simulink library "csu_kfo_kalman_filter_output_lib"  (R2015b)
settings: Solver=ode45  StartTime=0.0  StopTime=10.0  RelTol=1e-3
libraries: util_common_lib x4, util_info_lib x2
settings Model: Creator=escrane  LastModifiedBy=Mark Agbayani
settings DataIOCC: SaveFormat=Array
settings DebuggingCC: UnderspecifiedInitializationDetection=Classic  MergeDetectMultiDrivingBlocksExec=none  SolverPrmCheckMsg=warning  StateNameClashWarn=warning
settings HardwareCC: ProdBitPerPointer=32  ProdLargestAtomicFloat=None  ProdIntDivRoundTo=Undefined  ProdEndianess=Unspecified  ProdWordSize=32  ProdHWDeviceType=32-bit Generic
settings GRTTargetCC: GeneratePreprocessorConditionals=Disable all
settings ConfigComp: CovModelRefEnable=Off  CovSFcnEnable=off

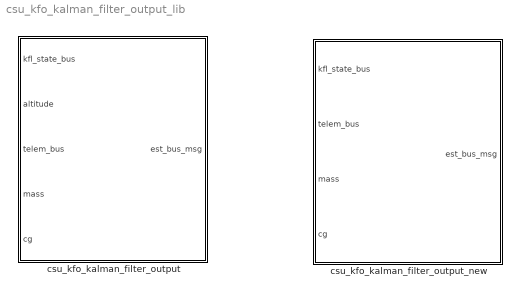
== system csu_kfo_kalman_filter_output_lib ==
  csu_kfo_kalman_filter_output : Subsystem
  csu_kfo_kalman_filter_output_new : Subsystem

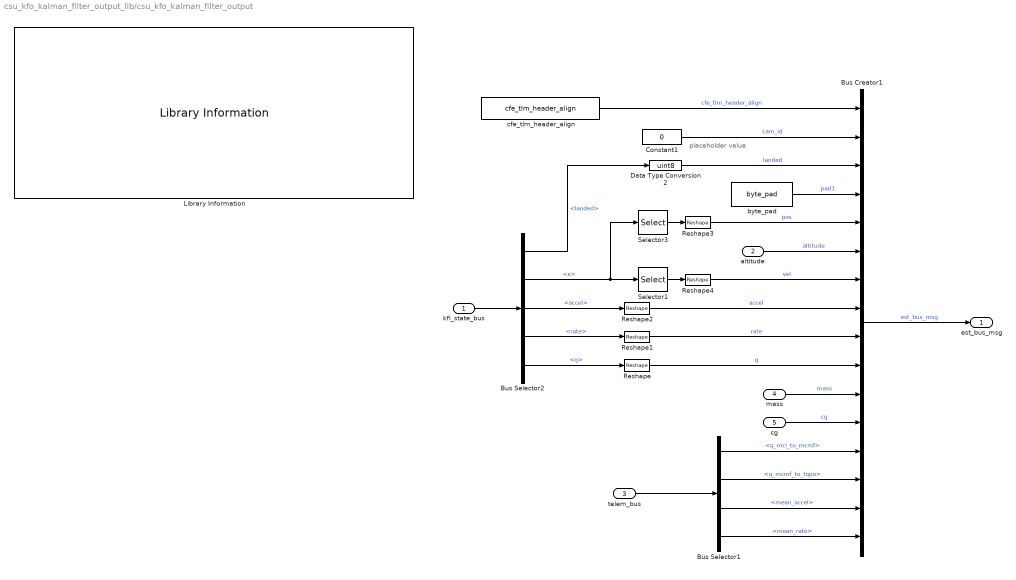
== system csu_kfo_kalman_filter_output_lib/csu_kfo_kalman_filter_output ==
  note: placeholder value
  kfl_state_bus : Inport
  altitude : Inport  Port=2
  telem_bus : Inport  Port=3
  mass : Inport  Port=4
  cg : Inport  Port=5
  Bus Creator1 : BusCreator  Inputs=16  OutDataTypeStr=Bus: est_bus_msg  NonVirtualBus=on
  Bus Selector1 : BusSelector  OutputSignals=q_mci_to_mcmf,q_mcmf_to_topo,mean_accel,mean_rate
  Bus Selector2 : BusSelector  OutputSignals=landed,x,accel,rate,q
  Constant1 : Constant  Value=0  OutDataTypeStr=uint8
  Data Type Conversion2 : DataTypeConversion  OutDataTypeStr=uint8
  Library Information : util_info_lib/Library Information  owner='escrane'
  Reshape{,1..4} (5 alike) : Reshape
  Selector1 : Selector  InputPortWidth=kfl_n_state  IndexOptions=Index vector (dialog)  Indices=kfl_vel_index  OutputSizes=1
  Selector3 : Selector  InputPortWidth=kfl_n_state  IndexOptions=Index vector (dialog)  Indices=kfl_pos_index  OutputSizes=1
  byte_pad : util_common_lib/byte_pad  n_bytes=2
  cfe_tlm_header_align : util_common_lib/cfe_tlm_header_align
  est_bus_msg : Outport
  wires:
  Bus Selector1/4 -> Bus Creator1/16  "<mean_rate>"
  Bus Selector1/3 -> Bus Creator1/15  "<mean_accel>"
  Bus Selector1/1 -> Bus Creator1/13  "<q_mci_to_mcmf>"
  Bus Selector1/2 -> Bus Creator1/14  "<q_mcmf_to_topo>"
  telem_bus/1 -> Bus Selector1/1
  cg/1 -> Bus Creator1/12  "cg"
  mass/1 -> Bus Creator1/11  "mass"
  kfl_state_bus/1 -> Bus Selector2/1
  cfe_tlm_header_align/1 -> Bus Creator1/1  "cfe_tlm_header_align"
  Bus Selector2/1 -> Data Type Conversion2/1  "<landed>"
  byte_pad/1 -> Bus Creator1/4  "pad1"
  Constant1/1 -> Bus Creator1/2  "cam_id"
  Reshape2/1 -> Bus Creator1/8  "accel"
  Bus Creator1/1 -> est_bus_msg/1  "est_bus_msg"
  Bus Selector2/5 -> Reshape/1  "<q>"
  Bus Selector2/4 -> Reshape1/1  "<rate>"
  Bus Selector2/3 -> Reshape2/1  "<accel>"
  Selector1/1 -> Reshape4/1
  Bus Selector2/2 -> Selector1/1, Selector3/1  "<x>"
  Reshape/1 -> Bus Creator1/10  "q"
  Reshape1/1 -> Bus Creator1/9  "rate"
  Reshape4/1 -> Bus Creator1/7  "vel"
  Reshape3/1 -> Bus Creator1/5  "pos"
  Selector3/1 -> Reshape3/1
  Data Type Conversion2/1 -> Bus Creator1/3  "landed"
  altitude/1 -> Bus Creator1/6  "altitude"

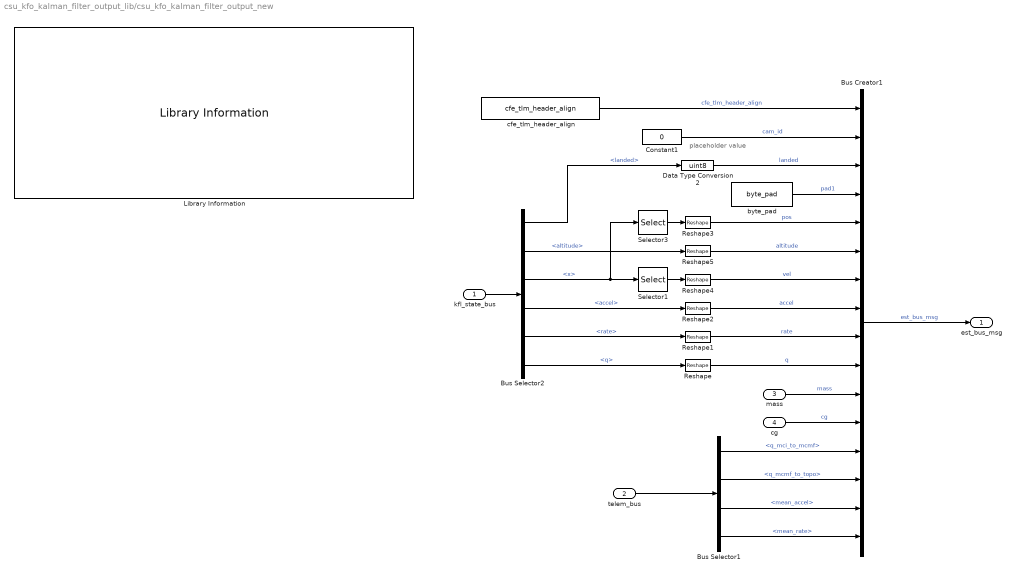
== system csu_kfo_kalman_filter_output_lib/csu_kfo_kalman_filter_output_new ==
  note: placeholder value
  kfl_state_bus : Inport
  telem_bus : Inport  Port=2
  mass : Inport  Port=3
  cg : Inport  Port=4
  Bus Creator1 : BusCreator  Inputs=16  OutDataTypeStr=Bus: est_bus_msg  NonVirtualBus=on
  Bus Selector1 : BusSelector  OutputSignals=q_mci_to_mcmf,q_mcmf_to_topo,mean_accel,mean_rate
  Bus Selector2 : BusSelector  OutputSignals=landed,altitude,x,accel,rate,q
  Constant1 : Constant  Value=0  OutDataTypeStr=uint8
  Data Type Conversion2 : DataTypeConversion  OutDataTypeStr=uint8
  Library Information : util_info_lib/Library Information  owner='escrane'
  Reshape{,1..5} (6 alike) : Reshape
  Selector1 : Selector  InputPortWidth=kfl_n_state  IndexOptions=Index vector (dialog)  Indices=kfl_vel_index  OutputSizes=1
  Selector3 : Selector  InputPortWidth=kfl_n_state  IndexOptions=Index vector (dialog)  Indices=kfl_pos_index  OutputSizes=1
  byte_pad : util_common_lib/byte_pad  n_bytes=2
  cfe_tlm_header_align : util_common_lib/cfe_tlm_header_align
  est_bus_msg : Outport
  wires:
  Reshape5/1 -> Bus Creator1/6  "altitude"
  Bus Selector1/4 -> Bus Creator1/16  "<mean_rate>"
  Bus Selector1/3 -> Bus Creator1/15  "<mean_accel>"
  Bus Selector1/1 -> Bus Creator1/13  "<q_mci_to_mcmf>"
  Bus Selector1/2 -> Bus Creator1/14  "<q_mcmf_to_topo>"
  telem_bus/1 -> Bus Selector1/1
  cg/1 -> Bus Creator1/12  "cg"
  mass/1 -> Bus Creator1/11  "mass"
  kfl_state_bus/1 -> Bus Selector2/1
  cfe_tlm_header_align/1 -> Bus Creator1/1  "cfe_tlm_header_align"
  Bus Selector2/1 -> Data Type Conversion2/1  "<landed>"
  byte_pad/1 -> Bus Creator1/4  "pad1"
  Constant1/1 -> Bus Creator1/2  "cam_id"
  Reshape2/1 -> Bus Creator1/8  "accel"
  Bus Creator1/1 -> est_bus_msg/1  "est_bus_msg"
  Bus Selector2/6 -> Reshape/1  "<q>"
  Bus Selector2/5 -> Reshape1/1  "<rate>"
  Bus Selector2/4 -> Reshape2/1  "<accel>"
  Selector1/1 -> Reshape4/1
  Bus Selector2/3 -> Selector1/1, Selector3/1  "<x>"
  Reshape/1 -> Bus Creator1/10  "q"
  Reshape1/1 -> Bus Creator1/9  "rate"
  Reshape4/1 -> Bus Creator1/7  "vel"
  Reshape3/1 -> Bus Creator1/5  "pos"
  Selector3/1 -> Reshape3/1
  Data Type Conversion2/1 -> Bus Creator1/3  "landed"
  Bus Selector2/2 -> Reshape5/1  "<altitude>"
